simulink model "simulink_experiments_PP_der"  (R2019b)
settings: Solver=ode1  StartTime=0.0  StopTime=inf  FixedStep=0.002  RelTol=1e-3  EnableMultiTasking=on
PostLoadFcn:
  | qc_set_target_type(getConfigSet(bdroot, 'QUARC Default Target Configuration'));
undefined symbols (not defined in the file): HIL, Kpp_int, Kpp_state, qc_get_step_size
libraries: quarc_library x4
settings Model: SimulationMode=external  ExtModeTrigDuration=5000  Creator=CFulford  LastModifiedBy=Student
settings SolverCC: PositivePriorityOrder=on
settings DataIOCC: LimitDataPoints=on  SaveFormat=Array  SignalLoggingSaveFormat=ModelDataLogs  ReturnWorkspaceOutputs=off
settings OptimizationCC: ExpressionDepthLimit=2147483647  InitFltsAndDblsToZero=on  LifeSpan=inf
settings DebuggingCC: SaveWithParameterizedLinksMsg=none  UnderspecifiedInitializationDetection=Classic  MergeDetectMultiDrivingBlocksExec=none  SolverPrmCheckMsg=warning  MultiTaskDSMMsg=warning  MultiTaskCondExecSysMsg=none  FcnCallInpInsideContextMsg=warning  StateNameClashWarn=warning  SFUnexpectedBacktrackingDiag=warning  SFNoUnconditionalDefaultTransitionDiag=warning  SFExecutionAtInitializationDiag=none  ArithmeticOperatorsInVariantConditions=warning
settings HardwareCC: ProdBitPerPointer=32  ProdBitPerSizeT=32  ProdBitPerPtrDiffT=32  ProdLargestAtomicFloat=None  ProdIntDivRoundTo=Undefined  ProdEndianess=Unspecified  ProdWordSize=32  ProdHWDeviceType=32-bit Generic
settings ModelReferenceCC: PropagateSignalLabelsOutOfModel=off
settings SFSimCC: SimUseLocalCustomCode=off  CustomCodeUndefinedFunction=UseInterfaceOnly
settings RTWCC: Description=QUARC Win64 Target  SystemTargetFile=quarc_win64.tlc  TemplateMakefile=quarc_default_tmf  RTWUseLocalCustomCode=off
settings CodeAppCC: StateflowObjectComments=on
settings STFCustomTargetCC: TargetPreCompLibLocation=C:\PROGRA~3\QUARC\lib\2019b\win64\release  ConcurrentExecutionCompliant=on  CombineOutputUpdateFcns=on  CPPClassGenCompliant=on  SystemTargetFile=quarc_win64.tlc
settings GRTTargetCC: TargetPreCompLibLocation=C:\PROGRA~3\QUARC\lib\2019b\win64\release  TargetLangStandard=C89/C90 (ANSI)  ParMdlRefBuildCompliant=off  CompOptLevelCompliant=off  MatFileLogging=off  UseToolchainInfoCompliant=off  ExtMode=on  ExtModeMexFile=quarc_comm
settings ConfigComp: CovMetricSettings=dw  CovSaveCumulativeToWorkspaceVar=on  CovSaveSingleToWorkspaceVar=on  CovExternalEMLEnable=off  CovSFcnEnable=off

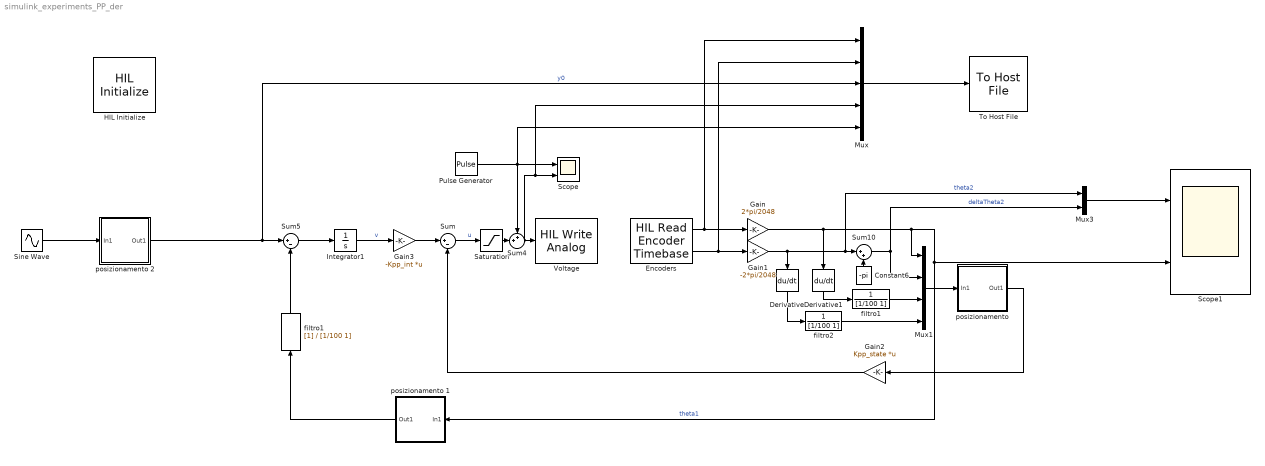
== system simulink_experiments_PP_der ==
  Constant6 : Constant  Value=-pi
  Derivative : Derivative
  Derivative1 : Derivative
  Encoders : quarc_library/Data Acquisition/Generic/Timebases/HIL Read Encoder Timebase  object_name=HIL-1  clock=0  channels=[0:1]  samples_in_buffer=max(ceil(1/qc_get_step_size), 1)  active=on  vector_output=off  data_type_mode=Inherit via back propagation  data_type=double
  Gain : Gain  Gain=2*pi/2048
  Gain1 : Gain  Gain=-2*pi/2048
  Gain2 : Gain  Gain=Kpp_state  Multiplication=Matrix(K*u)
  Gain3 : Gain  Gain=-Kpp_int  Multiplication=Matrix(K*u)
  HIL Initialize : quarc_library/Data Acquisition/Generic/Configuration/HIL Initialize  Priority=-99  object_name=HIL-1  board_type=qube_servo2_usb  board_number=0  board_options=""  exclusive=off  active=off  hardware_clocks=[0]  clock_modes=[]  initial_clock_frequencies=[]  set_clock_params_at_start=off  set_clock_params_at_switch_in=off  set_clock_frequencies_at_start=off  set_clock_frequencies_at_switch_in=off  analog_input_channels=[0]  analog_input_configurations=[]  analog_input_maximums=3  analog_input_minimums=-3  set_analog_input_params_at_start=off  set_analog_input_params_at_switch_in=off  analog_output_channels=[0]  analog_output_maximums=15  analog_output_minimums=-15  initial_analog_outputs=[0]  final_analog_outputs=[0]  watchdog_analog_outputs=0  set_analog_output_params_at_start=off  set_analog_output_params_at_switch_in=off  set_analog_outputs_at_start=on  set_analog_outputs_at_switch_in=off  set_analog_outputs_at_terminate=on  set_analog_outputs_at_switch_out=off  set_analog_outputs_on_watchdog=on  digital_input_channels=[]  digital_output_channels=[0]  digital_output_configuration=[]  initial_digital_outputs=[1]  final_digital_outputs=[0]  watchdog_digital_outputs=[0]  set_digital_output_params_at_start=off  set_digital_output_params_at_switch_in=off  set_digital_outputs_at_start=on  set_digital_outputs_at_switch_in=off  set_digital_outputs_at_terminate=on  set_digital_outputs_at_switch_out=off  set_digital_outputs_on_watchdog=on  encoder_channels=[0:1]  quadrature=[4]  encoder_filter_frequency=[]  initial_encoder_counts=[0]  set_encoder_params_at_start=off  set_encoder_params_at_switch_in=off  set_encoder_counts_at_start=on  set_encoder_counts_at_switch_in=off  pwm_channels=[]  pwm_modes=[]  pwm_frequency=[]  pwm_configuration=[]  pwm_alignment=[]  pwm_polarity=[]  pwm_leading_deadband=[]  pwm_trailing_deadband=[]  initial_pwm_outputs=[]  final_pwm_outputs=[]  watchdog_pwm_outputs=[]  set_pwm_params_at_start=off  set_pwm_params_at_switch_in=off  set_pwm_outputs_at_start=off  set_pwm_outputs_at_switch_in=off  set_pwm_outputs_at_terminate=off  set_pwm_outputs_at_switch_out=off  set_pwm_outputs_on_watchdog=off  other_output_channels=[11000:11002]  initial_other_outputs=[0 1 0]  final_other_outputs=[1 0 0]  watchdog_other_outputs=[0 0 1]  set_other_outputs_at_start=on  set_other_outputs_at_switch_in=off  set_other_outputs_at_terminate=on  set_other_outputs_at_switch_out=off  set_other_outputs_on_watchdog=on
  Integrator1 : Integrator
  Mux : Mux  Inputs=5
  Mux1 : Mux
  Mux3 : Mux  Inputs=2
  Pulse Generator : DiscretePulseGenerator  PulseType=Time based  Amplitude=0  Period=10
  Saturation : Saturate  UpperLimit=10  LowerLimit=-10
  Scope : Scope  NumInputPorts=2
  Scope1 : Scope  NumInputPorts=2
  Sine Wave : Sin  Amplitude=0.8  Frequency=0.5  SampleTime=0
  Sum : Sum  Inputs=|+-
  Sum10 : Sum  Inputs=|++
  Sum4 : Sum  Inputs=++|
  Sum5 : Sum  Inputs=|+-
  To Host File : quarc_library/Sinks/To Host/To Host File  file_name=data_%{date}_%{time}.mat  variable_name=data_%{date}_%{time}  decimation=1  sample_time=-1  file_format=MAT-file v.5  options=No header or footer  append=off  final_file_name=data_28-May-2024_17-30-13.mat  bitrate=2000000
  Voltage : quarc_library/Data Acquisition/Generic/Immediate I//O/HIL Write Analog  object_name=HIL-1  channels=0  sample_time=-1  active=off  vector_input=off
  filtro1 : TransferFcn  Denominator=[1/100 1]
  "filtro1 " : TransferFcn  Denominator=[1/100 1]
  filtro2 : TransferFcn  Denominator=[1/100 1]
  "posizionamento " : Subsystem
  posizionamento 1 : Subsystem
  posizionamento 2 : Subsystem
  wires:
  Mux/1 -> To Host File/1
  Constant6/1 -> Sum10/2
  Sum10/1 -> Mux1/2, Mux3/2  "deltaTheta2"
  Gain2/1 -> Sum/2
  Encoders/2 -> Gain1/1, Mux/2
  Encoders/1 -> Gain/1, Mux/1
  Integrator1/1 -> Gain3/1  "v"
  Sum/1 -> Saturation/1  "u"
  Sum5/1 -> Integrator1/1
  "filtro1 "/1 -> Mux1/3
  Derivative1/1 -> "filtro1 "/1
  Derivative/1 -> filtro2/1
  filtro2/1 -> Mux1/4
  Gain1/1 -> Mux3/1, Sum10/1, Derivative/1  "theta2"
  Gain/1 -> posizionamento 1/1(In1), Scope1/2, Mux1/1, Derivative1/1  "theta1"
  posizionamento 2/1(Out1) -> Mux/3, Sum5/1  "y0"
  Mux3/1 -> Scope1/1
  Mux1/1 -> "posizionamento "/1(In1)
  "posizionamento "/1(Out1) -> Gain2/1
  posizionamento 1/1(Out1) -> filtro1/1
  Gain3/1 -> Sum/1
  Saturation/1 -> Sum4/2
  Pulse Generator/1 -> Mux/5, Scope/1, Sum4/1
  Sum4/1 -> Mux/4, Scope/2, Voltage/1
  filtro1/1 -> Sum5/2
  Sine Wave/1 -> posizionamento 2/1(In1)

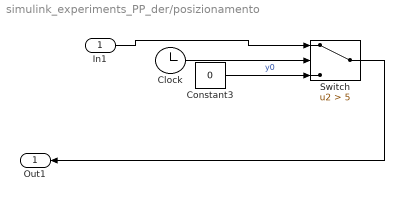
== system simulink_experiments_PP_der/posizionamento  ==
  In1 : Inport
  Clock : Clock
  Constant3 : Constant  Value=0
  Switch : Switch  Criteria=u2 > Threshold  Threshold=5
  Out1 : Outport
  wires:
  In1/1 -> Switch/1
  Constant3/1 -> Switch/3  "y0"
  Clock/1 -> Switch/2
  Switch/1 -> Out1/1

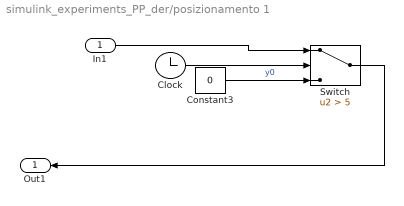
== system simulink_experiments_PP_der/posizionamento 1 ==
  In1 : Inport
  Clock : Clock
  Constant3 : Constant  Value=0
  Switch : Switch  Criteria=u2 > Threshold  Threshold=5
  Out1 : Outport
  wires:
  In1/1 -> Switch/1
  Constant3/1 -> Switch/3  "y0"
  Clock/1 -> Switch/2
  Switch/1 -> Out1/1

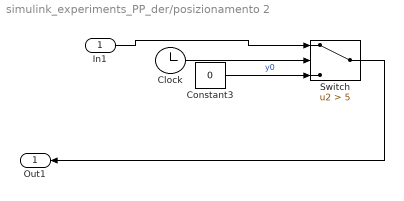
== system simulink_experiments_PP_der/posizionamento 2 ==
  In1 : Inport
  Clock : Clock
  Constant3 : Constant  Value=0
  Switch : Switch  Criteria=u2 > Threshold  Threshold=5
  Out1 : Outport
  wires:
  In1/1 -> Switch/1
  Constant3/1 -> Switch/3  "y0"
  Clock/1 -> Switch/2
  Switch/1 -> Out1/1
